simulink model "Project"  (R2018a)
settings: Solver=VariableStepAuto  StartTime=0  StopTime=1  FixedStep=Ts  RelTol=1e-3  AbsTol=1e-3
PreLoadFcn:
  | Ts=2e-6;
  | Ts_Control=100e-6;
undefined symbols (not defined in the file): Hydride, Metal, Nickel, Vnom_dc
libraries: powerlib x111, powerlib_extras x45, simulink x32, powerlib_meascontrol x13, dspswit3 x9, electricdrivelib x2, re_lib x2
(part 2 of 4)

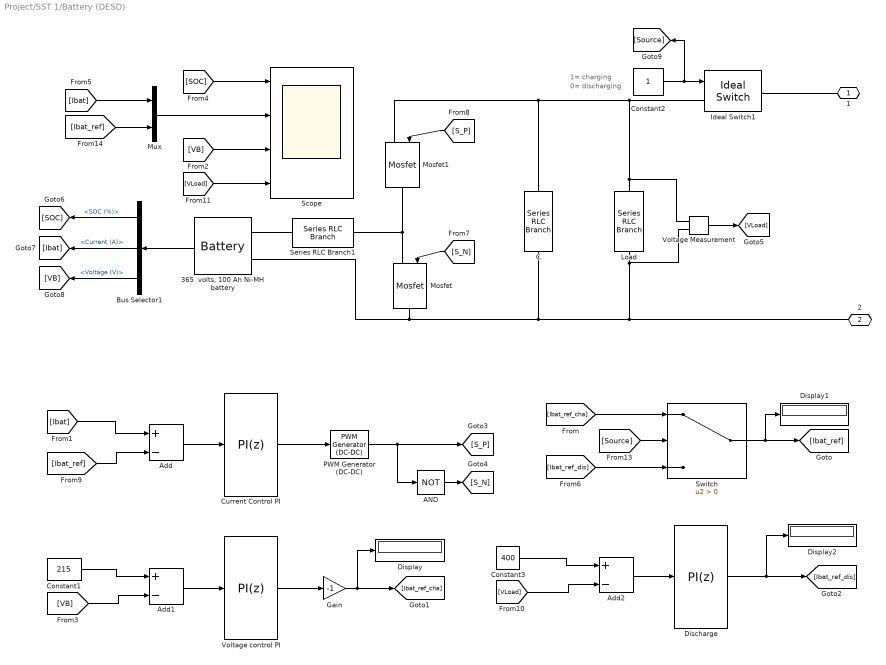
== system Project/SST 1/Battery (DESD) ==
  note: 1= charging
  note: 0= discharging
  "365  volts, 100 Ah Ni-MH battery" : electricdrivelib/Extra Sources/Battery  BatType=Nickel-Metal-Hydride  ShowTempParam=off  ThermalPreset=no  ShowAgeParam=off  NomV=365  NomQ=100  SOC=45  Batt_Tr=1  PresetModel=on  MaxQ=107.6923  MinV=273.75  FullV=429.9576  Dis_rate=20  R=0.0365  Normal_OP=96.1538  expZone="[395.9322            20]"  current=[6.5 13 32.5]  Units=Time  Tci=20  NomT=25  T2=0  MaxQ2=2.208  FullV2=3.45  Normal_OP2=2.8  expZone2="[3.22        0.23]"  Rca=0.6  ti=1000  Dp=0  Neq0=0  Tsim=1e6  Ta1=25  Qeol=5.4*0.9  Reol=0.013333*1.2  Char_age=[2.3478, 3]  Dis_age=[2.3478, 10]  N1=1500  N2=10500  N3=1000  N4=1400  Ta2=45  N5=950
      settings: SourceProductName=Simscape Electrical
  AND : Logic  Operator=NOT  AllPortsSameDT=off  OutDataTypeStr=boolean
  Add : Sum  Inputs=+-
  Add1 : Sum  Inputs=+-
  Add2 : Sum  Inputs=+-
  Bus Selector1 : BusSelector  OutputSignals=SOC (%),Current (A),Voltage (V)
  C : powerlib/Elements/Series RLC Branch  LConnTagsString=__new0  RConnTagsString=__new0  BranchType=RC  Resistance=0  Inductance=1e-3  SetiL0=off  InitialCurrent=0  Capacitance=1000e-6  Setx0=off  InitialVoltage=0  Measurements=None
      settings: SourceProductName=Simscape Electrical
  Constant1 : Constant  Value=215
  Constant2 : Constant
  Constant3 : Constant  Value=400
  Current Control PI : simulink/Continuous/PID Controller  Controller=PI  TimeDomain=Discrete-time  SampleTime=50e-6  IntegratorMethod=Forward Euler  FilterMethod=Forward Euler  Form=Parallel  UseFilter=on  ControllerParametersSource=internal  P=0.005  I=10  D=0  N=100  InitialConditionSource=internal  InitialConditionForIntegrator=0.54  InitialConditionForFilter=0  ExternalReset=none  LimitOutput=on  UpperSaturationLimit=0.95  LowerSaturationLimit=0  LinearizeAsGain=off  AntiWindupMode=none  Kb=1  TrackingMode=off  Kt=1  PParamMin=[]  PParamMax=[]  IParamMin=[]  IParamMax=[]  DParamMin=[]  DParamMax=[]  NParamMin=[]  NParamMax=[]  KbParamMin=[]  KbParamMax=[]  KtParamMin=[]  KtParamMax=[]  POutMin=[]  POutMax=[]  IOutMin=[]  IOutMax=[]  DOutMin=[]  DOutMax=[]  NOutMin=[]  NOutMax=[]  KbOutMin=[]  KbOutMax=[]  KtOutMin=[]  KtOutMax=[]  IntegratorOutMin=[]  IntegratorOutMax=[]  FilterOutMin=[]  FilterOutMax=[]  SumOutMin=[]  SumOutMax=[]  SumI1OutMin=[]  SumI1OutMax=[]  SumI2OutMin=[]  SumI2OutMax=[]  SumI3OutMin=[]  SumI3OutMax=[]  SumDOutMin=[]  SumDOutMax=[]  SaturationOutMin=[]  SaturationOutMax=[]  IntegratorContinuousStateAttributes=''  IntegratorStateMustResolveToSignalObject=off  IntegratorRTWStateStorageClass=Auto  FilterContinuousStateAttributes=''  FilterStateMustResolveToSignalObject=off  FilterRTWStateStorageClass=Auto  DifferentiatorICPrevScaledInput=0  DifferentiatorOutMin=[]  DifferentiatorOutMax=[]  FilterDiffOutCoefMin=[]  FilterDiffOutCoefMax=[]  SumDenOutMin=[]  SumDenOutMax=[]  SumNumOutMin=[]  SumNumOutMax=[]  ReciprocalOutMin=[]  ReciprocalOutMax=[]  DivideOutMin=[]  DivideOutMax=[]  TunerSelectOption=Transfer Function Based (PID Tuner App)
  Discharge : simulink/Continuous/PID Controller  Controller=PI  TimeDomain=Discrete-time  SampleTime=50e-6  IntegratorMethod=Forward Euler  FilterMethod=Forward Euler  Form=Parallel  UseFilter=on  ControllerParametersSource=internal  P=0.25  I=50  D=0  N=100  InitialConditionSource=internal  InitialConditionForIntegrator=0  InitialConditionForFilter=0  ExternalReset=none  LimitOutput=on  UpperSaturationLimit=12  LowerSaturationLimit=0  LinearizeAsGain=off  AntiWindupMode=none  Kb=1  TrackingMode=off  Kt=1  PParamMin=[]  PParamMax=[]  IParamMin=[]  IParamMax=[]  DParamMin=[]  DParamMax=[]  NParamMin=[]  NParamMax=[]  KbParamMin=[]  KbParamMax=[]  KtParamMin=[]  KtParamMax=[]  POutMin=[]  POutMax=[]  IOutMin=[]  IOutMax=[]  DOutMin=[]  DOutMax=[]  NOutMin=[]  NOutMax=[]  KbOutMin=[]  KbOutMax=[]  KtOutMin=[]  KtOutMax=[]  IntegratorOutMin=[]  IntegratorOutMax=[]  FilterOutMin=[]  FilterOutMax=[]  SumOutMin=[]  SumOutMax=[]  SumI1OutMin=[]  SumI1OutMax=[]  SumI2OutMin=[]  SumI2OutMax=[]  SumI3OutMin=[]  SumI3OutMax=[]  SumDOutMin=[]  SumDOutMax=[]  SaturationOutMin=[]  SaturationOutMax=[]  IntegratorContinuousStateAttributes=''  IntegratorStateMustResolveToSignalObject=off  IntegratorRTWStateStorageClass=Auto  FilterContinuousStateAttributes=''  FilterStateMustResolveToSignalObject=off  FilterRTWStateStorageClass=Auto  DifferentiatorICPrevScaledInput=0  DifferentiatorOutMin=[]  DifferentiatorOutMax=[]  FilterDiffOutCoefMin=[]  FilterDiffOutCoefMax=[]  SumDenOutMin=[]  SumDenOutMax=[]  SumNumOutMin=[]  SumNumOutMax=[]  ReciprocalOutMin=[]  ReciprocalOutMax=[]  DivideOutMin=[]  DivideOutMax=[]  TunerSelectOption=Transfer Function Based (PID Tuner App)
  Display : Display
  Display1 : Display
  Display2 : Display
  Gain : Gain  Gain=-1
  Ideal Switch1 : powerlib/Power Electronics/Ideal Switch  Ron=0.001  Lon=0  IC=0  Rs=1e5  Cs=inf  Measurements=off
      settings: SourceProductName=Simscape Electrical
  Load : powerlib/Elements/Series RLC Branch  LConnTagsString=__new0  RConnTagsString=__new0  BranchType=R  Resistance=10  Inductance=1e-3  SetiL0=off  InitialCurrent=0  Capacitance=1e-6  Setx0=off  InitialVoltage=0  Measurements=None
      settings: SourceProductName=Simscape Electrical
  Mosfet : powerlib/Power Electronics/Mosfet  Ron=0.1  Lon=0  Rd=0.01  Vfd=0  IC=0  Rs=1e5  Cs=inf  Measurements=off
      settings: SourceProductName=Simscape Electrical
  Mosfet1 : powerlib/Power Electronics/Mosfet  Ron=0.1  Lon=0  Rd=0.01  Vfd=0  IC=0  Rs=1e5  Cs=inf  Measurements=off
      settings: SourceProductName=Simscape Electrical
  Mux : Mux  Inputs=2
  PWM Generator (DC-DC) : powerlib_meascontrol/Pulse & Signal Generators/PWM Generator (DC-DC)  Fsw=10e3  Ts=5e-6
      settings: SourceProductName=Simscape Electrical
  Scope : Scope  NumInputPorts=4
  Series RLC Branch1 : powerlib/Elements/Series RLC Branch  LConnTagsString=__new0  RConnTagsString=__new0  BranchType=RL  Resistance=0.05  Inductance=5.76e-4  SetiL0=off  InitialCurrent=0  Capacitance=1e-6  Setx0=off  InitialVoltage=0  Measurements=None
      settings: SourceProductName=Simscape Electrical
  Switch : Switch  Criteria=u2 > Threshold
  Voltage Measurement : powerlib/Measurements/Voltage Measurement  PhasorSimulation=off  OutputType=Complex  PSBequivalent=0
      settings: SourceProductName=Simscape Electrical
  Voltage control PI : simulink/Continuous/PID Controller  Controller=PI  TimeDomain=Discrete-time  SampleTime=500e-6  IntegratorMethod=Forward Euler  FilterMethod=Forward Euler  Form=Parallel  UseFilter=on  ControllerParametersSource=internal  P=40  I=2000  D=0  N=100  InitialConditionSource=internal  InitialConditionForIntegrator=0  InitialConditionForFilter=0  ExternalReset=none  LimitOutput=on  UpperSaturationLimit=12  LowerSaturationLimit=0  LinearizeAsGain=off  AntiWindupMode=none  Kb=1  TrackingMode=off  Kt=1  PParamMin=[]  PParamMax=[]  IParamMin=[]  IParamMax=[]  DParamMin=[]  DParamMax=[]  NParamMin=[]  NParamMax=[]  KbParamMin=[]  KbParamMax=[]  KtParamMin=[]  KtParamMax=[]  POutMin=[]  POutMax=[]  IOutMin=[]  IOutMax=[]  DOutMin=[]  DOutMax=[]  NOutMin=[]  NOutMax=[]  KbOutMin=[]  KbOutMax=[]  KtOutMin=[]  KtOutMax=[]  IntegratorOutMin=[]  IntegratorOutMax=[]  FilterOutMin=[]  FilterOutMax=[]  SumOutMin=[]  SumOutMax=[]  SumI1OutMin=[]  SumI1OutMax=[]  SumI2OutMin=[]  SumI2OutMax=[]  SumI3OutMin=[]  SumI3OutMax=[]  SumDOutMin=[]  SumDOutMax=[]  SaturationOutMin=[]  SaturationOutMax=[]  IntegratorContinuousStateAttributes=''  IntegratorStateMustResolveToSignalObject=off  IntegratorRTWStateStorageClass=Auto  FilterContinuousStateAttributes=''  FilterStateMustResolveToSignalObject=off  FilterRTWStateStorageClass=Auto  DifferentiatorICPrevScaledInput=0  DifferentiatorOutMin=[]  DifferentiatorOutMax=[]  FilterDiffOutCoefMin=[]  FilterDiffOutCoefMax=[]  SumDenOutMin=[]  SumDenOutMax=[]  SumNumOutMin=[]  SumNumOutMax=[]  ReciprocalOutMin=[]  ReciprocalOutMax=[]  DivideOutMin=[]  DivideOutMax=[]  TunerSelectOption=Transfer Function Based (PID Tuner App)
  1 : PMIOPort  Side=Right
  2 : PMIOPort  Port=2  Side=Left
  wires:
  Current Control PI/1 -> PWM Generator (DC-DC)/1
  PWM Generator (DC-DC)/1 -> AND/1, [S_P]
  Bus Selector1/2 -> [Ibat]  "<Current (A)>"
  [SOC] -> Scope/1
  [S_N] -> Mosfet/1
  Discharge/1 -> Display2/1, [Ibat_ref_dis]
  [Ibat] -> Mux/1
  [Ibat_ref] -> Mux/2
  [VB] -> Add1/2
  "365  volts, 100 Ah Ni-MH battery"/1 -> Bus Selector1/1
  [VB] -> Scope/3
  Constant2/1 -> [Source], Ideal Switch1/1
  Bus Selector1/1 -> [SOC]  "<SOC (%)>"
  Add1/1 -> Voltage control PI/1
  Gain/1 -> Display/1, [Ibat_ref_cha]
  [S_P] -> Mosfet1/1
  [Ibat_ref_dis] -> Switch/3
  Voltage control PI/1 -> Gain/1
  [Ibat_ref] -> Add/2
  [Ibat] -> Add/1
  [VLoad] -> Add2/2
  Bus Selector1/3 -> [VB]  "<Voltage (V)>"
  Add/1 -> Current Control PI/1
  [VLoad] -> Scope/4
  Switch/1 -> [Ibat_ref], Display1/1
  Constant3/1 -> Add2/1
  AND/1 -> [S_N]
  [Source] -> Switch/2
  Mux/1 -> Scope/2
  Constant1/1 -> Add1/1
  [Ibat_ref_cha] -> Switch/1
  Add2/1 -> Discharge/1
  Voltage Measurement/1 -> [VLoad]
  connections:
  Ideal Switch1/LConn1 -- Load/RConn1 -- Voltage Measurement/LConn1 -- Mosfet1/LConn1 -- C/RConn1
  Load/LConn1 -- 2/RConn1 -- "365  volts, 100 Ah Ni-MH battery"/LConn2 -- Mosfet/RConn1 -- C/LConn1 -- Voltage Measurement/LConn2
  Series RLC Branch1/RConn1 -- Mosfet1/RConn1 -- Mosfet/LConn1
  "365  volts, 100 Ah Ni-MH battery"/LConn1 -- Series RLC Branch1/LConn1
  Ideal Switch1/RConn1 -- 1/RConn1

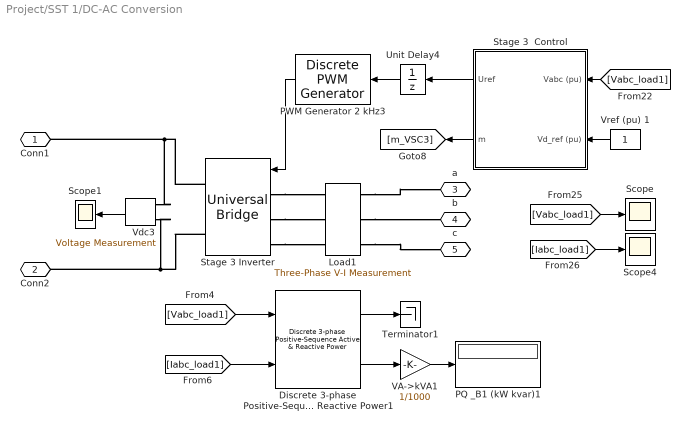
== system Project/SST 1/DC-AC Conversion ==
  Discrete 3-phase Positive-Sequence Active & Reactive Power1 : powerlib_extras/Discrete Measurements/Discrete 3-phase  Positive-Sequence  Active & Reactive Power  Freq=60  Par_Vinit=[0 0]  Par_Iinit=[0 0]  Ts=Ts
  Load1 : powerlib/Measurements/Three-Phase V-I Measurement  VoltageMeasurement=phase-to-phase  SetLabelV=on  LabelV=Vabc_load1  Vpu=off  VpuLL=off  CurrentMeasurement=yes  SetLabelI=on  LabelI=Iabc_load1  Ipu=off  Pbase=1e3  Vbase=380  OutputType=Magnitude  PhasorSimulation=off  PSBequivalent=0
  PQ _B1 (kW kvar)1 : Display
      settings: Decimation=2000
  PWM Generator 2 kHz3 : powerlib_extras/Discrete  Control Blocks/Discrete PWM Generator  GeneratorMode="3-arm  bridge (6 pulses)"  Fc=2000  Ts=Ts  Internal=off  mIndex=0.4  Freq=60  Phase=0
  Scope : Scope
  Scope1 : Scope
  Scope4 : Scope
  Stage 3 Inverter : powerlib/Power Electronics/Universal Bridge  Arms=3  SnubberResistance=1e5  SnubberCapacitance=inf  Device=IGBT / Diodes  Ron=1e-3  Lon=0  ForwardVoltages="[  0.0  0.0  ]"  ForwardVoltage=.8  GTOparameters=[ 1e-6 ,1e-6 ]  IGBTparameters="[ 0  0 ]"  Measurements=Device currents  Measurements_2=None  converterType=Rectifier
  "Stage 3  Control " : Subsystem  mask(Voltage Regulator){Kp=0.3, Ki=300, Vnom_load=380, Vnom_dc=680, Ts=Ts_Control}
      mask prompts: Kp "Proportional gain  Kp:"; Ki "Integral gain Ki:"; Vnom_load "Nominal load voltage (VrmsLL)"; Vnom_dc "Nominal DC bus voltage (V):"; Ts "Sample time (s) :"
  Terminator1 : Terminator
  Unit Delay4 : UnitDelay  SampleTime=Ts_Control
  VA->kVA1 : Gain  Gain=1/1000
  "Vdc3 " : powerlib/Measurements/Voltage Measurement  PhasorSimulation=off  OutputType=Complex  PSBequivalent=0
  Vref (pu) 1 : Constant
  Conn1 : PMIOPort  Side=Right
  Conn2 : PMIOPort  Port=2  Side=Right
  a : PMIOPort  Tag=PMCPort  Port=3  Side=Left
  " b" : PMIOPort  Tag=PMCPort  Port=4  Side=Left
  " c" : PMIOPort  Tag=PMCPort  Port=5  Side=Left
  wires:
  "Stage 3  Control "/2(m) -> [m_VSC3]
  Vref (pu) 1/1 -> "Stage 3  Control "/2(Vd_ref (pu))
  [Vabc_load1] -> "Stage 3  Control "/1(Vabc (pu))
  [Vabc_load1] -> Discrete 3-phase Positive-Sequence Active & Reactive Power1/1
  PWM Generator 2 kHz3/1 -> Stage 3 Inverter/1
  Unit Delay4/1 -> PWM Generator 2 kHz3/1
  VA->kVA1/1 -> PQ _B1 (kW kvar)1/1
  [Iabc_load1] -> Discrete 3-phase Positive-Sequence Active & Reactive Power1/2
  "Stage 3  Control "/1(Uref) -> Unit Delay4/1
  [Iabc_load1] -> Scope4/1
  [Vabc_load1] -> Scope/1
  Discrete 3-phase Positive-Sequence Active & Reactive Power1/2 -> VA->kVA1/1
  Discrete 3-phase Positive-Sequence Active & Reactive Power1/1 -> Terminator1/1
  "Vdc3 "/1 -> Scope1/1
  connections:
  Load1/RConn2 -- " b"/RConn1
  Load1/RConn3 -- " c"/RConn1
  Load1/RConn1 -- a/RConn1
  Stage 3 Inverter/LConn1 -- Load1/LConn1
  Stage 3 Inverter/LConn2 -- Load1/LConn2
  Stage 3 Inverter/LConn3 -- Load1/LConn3
  Stage 3 Inverter/RConn2 -- "Vdc3 "/LConn2 -- Conn2/RConn1
  Stage 3 Inverter/RConn1 -- "Vdc3 "/LConn1 -- Conn1/RConn1

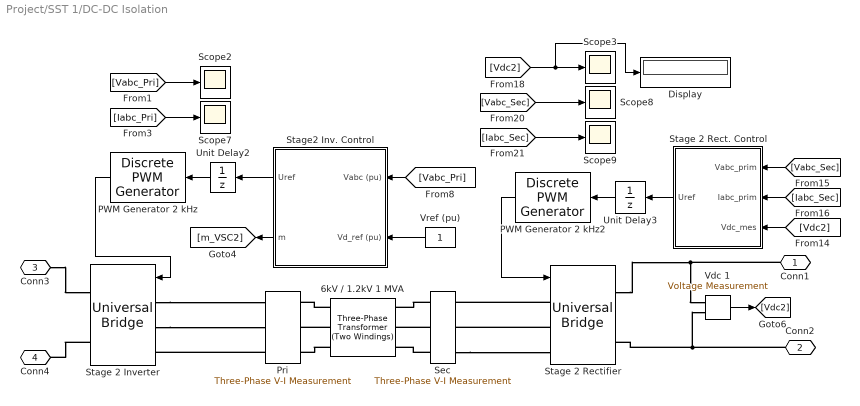
== system Project/SST 1/DC-DC Isolation ==
  6kV / 1.2kV 1 MVA : powerlib/Elements/Three-Phase Transformer (Two Windings)  Winding1Connection=Yg  Winding2Connection=Yg  CoreType=Three single-phase transformers  SetSaturation=off  Hysteresis=off  DataFile='hysteresis'  SetInitialFlux=off  Measurements=None  UNITS=pu  NominalPower=[ 1e6 , 60 ]  Winding1=[ 6e3 , 0.004 , 0.02 ]  Winding2=[ 1.2e3 , 0.004 , 0.02 ]  Rm=200  Lm=200  L0=0.5  Saturation="[ 0,0  ;  0.005,1.2  ;  1.0,1.4 ]"  InitialFluxes=[ 0.8 , -0.8 , 0.7 ]  MoreParameters=off  BreakLoop=off  DataType=off  TransfoNumber=0
  Display : Display
  PWM Generator 2 kHz : powerlib_extras/Discrete  Control Blocks/Discrete PWM Generator  GeneratorMode="3-arm  bridge (6 pulses)"  Fc=2000  Ts=Ts  Internal=off  mIndex=0.4  Freq=60  Phase=0
  PWM Generator 2 kHz2 : powerlib_extras/Discrete  Control Blocks/Discrete PWM Generator  GeneratorMode="3-arm  bridge (6 pulses)"  Fc=2000  Ts=Ts  Internal=off  mIndex=0.4  Freq=60  Phase=0
  Pri : powerlib/Measurements/Three-Phase V-I Measurement  VoltageMeasurement=phase-to-ground  SetLabelV=on  LabelV=Vabc_Pri  Vpu=off  VpuLL=off  CurrentMeasurement=yes  SetLabelI=on  LabelI=Iabc_Pri  Ipu=off  Pbase=1e3  Vbase=380  OutputType=Magnitude  PhasorSimulation=off  PSBequivalent=0
  Scope{2..3,7..9} (5 alike) : Scope
  Sec : powerlib/Measurements/Three-Phase V-I Measurement  VoltageMeasurement=phase-to-ground  SetLabelV=on  LabelV=Vabc_Sec  Vpu=off  VpuLL=off  CurrentMeasurement=yes  SetLabelI=on  LabelI=Iabc_Sec  Ipu=off  Pbase=100e6  Vbase=500e3  OutputType=Magnitude  PhasorSimulation=off  PSBequivalent=0
  Stage 2 Inverter : powerlib/Power Electronics/Universal Bridge  Arms=3  SnubberResistance=1e5  SnubberCapacitance=inf  Device=IGBT / Diodes  Ron=1e-3  Lon=0  ForwardVoltages="[  0.0  0.0  ]"  ForwardVoltage=.8  GTOparameters=[ 1e-6 ,1e-6 ]  IGBTparameters="[ 0  0 ]"  Measurements=None  Measurements_2=None  converterType=Rectifier
  Stage 2 Rectifier : powerlib/Power Electronics/Universal Bridge  Arms=3  SnubberResistance=1e5  SnubberCapacitance=inf  Device=IGBT / Diodes  Ron=1e-3  Lon=0  ForwardVoltages="[  0  0  ]"  ForwardVoltage=0  GTOparameters=[ 10e-6 , 20e-6 ]  IGBTparameters="[ 0  0  ]"  Measurements=None  Measurements_2=None  converterType=Rectifier
  Stage 2 Rect. Control : Subsystem  mask(VSC Main Controller){nom=[ 50e3  60 ], Vnom=[ 1.6e3 400 ], Vnom_dc=680, RLxfo=[0.008  0.04 ], RLchoke=[2e-3*(2*pi*60)/50   2e-3], K_VDCreg=[7  800], K_Ireg=[0.3 20]*1.5, Ts=Ts_Control}
      mask prompts: nom "Nominal power and frequency [ Pnom(VA)  Fnom(Hz) ]:"; Vnom "Nominal primary and secondary voltages (Vrms LL) [ Vnom_prim   Vnom_sec ]:"; Vnom_dc "Nominal DC bus voltage (V):"; RLxfo "Total transformer leakage impedance (pu/Pnom) [ Rxfo  Lxf ]"; RLchoke "Choke impedance [ R(ohm) L(H) ]"; K_VDCreg "VDC regultator gains [ Kp  Ki ]:"; K_Ireg "Current regulator gains [ Kp  Ki ]:"; Ts "Sample time"
      mask init: same as Project/SST 1/AC-DC Conversion/Stage1 Control
  "Stage2 Inv. Control " : Subsystem  mask(Voltage Regulator){Kp=0.3, Ki=300, Vnom_load=3.5e3, Vnom_dc=680, Ts=Ts_Control}
      mask prompts: Kp "Proportional gain  Kp:"; Ki "Integral gain Ki:"; Vnom_load "Nominal load voltage (VrmsLL)"; Vnom_dc "Nominal DC bus voltage (V):"; Ts "Sample time (s) :"
  Unit Delay2 : UnitDelay  SampleTime=Ts_Control
  Unit Delay3 : UnitDelay  SampleTime=Ts_Control
  Vdc 1 : powerlib/Measurements/Voltage Measurement  Tag=PoWeRsYsTeMmEaSuReMeNt  PhasorSimulation=off  OutputType=Magnitude  PSBequivalent=0
  "Vref (pu) " : Constant
  Conn1 : PMIOPort  Side=Left
  Conn2 : PMIOPort  Port=2  Side=Left
  Conn3 : PMIOPort  Port=3  Side=Right
  Conn4 : PMIOPort  Port=4  Side=Right
  wires:
  "Vref (pu) "/1 -> "Stage2 Inv. Control "/2(Vd_ref (pu))
  [Vdc2] -> Stage 2 Rect. Control/3(Vdc_mes)
  [Iabc_Sec] -> Scope9/1
  PWM Generator 2 kHz/1 -> Stage 2 Inverter/1
  Vdc 1/1 -> [Vdc2]
  [Vabc_Pri] -> Scope2/1
  [Iabc_Pri] -> Scope7/1
  [Vdc2] -> Display/1, Scope3/1
  [Vabc_Sec] -> Scope8/1
  "Stage2 Inv. Control "/2(m) -> [m_VSC2]
  PWM Generator 2 kHz2/1 -> Stage 2 Rectifier/1
  Stage 2 Rect. Control/1(Uref) -> Unit Delay3/1
  [Vabc_Pri] -> "Stage2 Inv. Control "/1(Vabc (pu))
  Unit Delay3/1 -> PWM Generator 2 kHz2/1
  [Vabc_Sec] -> Stage 2 Rect. Control/1(Vabc_prim)
  [Iabc_Sec] -> Stage 2 Rect. Control/2(Iabc_prim)
  "Stage2 Inv. Control "/1(Uref) -> Unit Delay2/1
  Unit Delay2/1 -> PWM Generator 2 kHz/1
  connections:
  Stage 2 Inverter/LConn2 -- Pri/LConn2
  Sec/LConn1 -- 6kV / 1.2kV 1 MVA/RConn1
  6kV / 1.2kV 1 MVA/LConn2 -- Pri/RConn2
  Stage 2 Rectifier/RConn2 -- Vdc 1/LConn2 -- Conn2/RConn1
  Stage 2 Inverter/LConn1 -- Pri/LConn1
  Stage 2 Rectifier/RConn1 -- Vdc 1/LConn1 -- Conn1/RConn1
  6kV / 1.2kV 1 MVA/LConn3 -- Pri/RConn3
  Sec/LConn2 -- 6kV / 1.2kV 1 MVA/RConn2
  6kV / 1.2kV 1 MVA/LConn1 -- Pri/RConn1
  Sec/LConn3 -- 6kV / 1.2kV 1 MVA/RConn3
  Pri/LConn3 -- Stage 2 Inverter/LConn3
  Stage 2 Inverter/RConn2 -- Conn4/RConn1
  Conn3/RConn1 -- Stage 2 Inverter/RConn1
  Sec/RConn3 -- Stage 2 Rectifier/LConn3
  Stage 2 Rectifier/LConn1 -- Sec/RConn1
  Stage 2 Rectifier/LConn2 -- Sec/RConn2

== system Project/SST 1/PV (DRER) ==
  Bus Selector1 : BusSelector  OutputSignals=V_PV,I_PV,I_diode
  C1 : powerlib/Elements/Series RLC Branch  LConnTagsString=__new0  RConnTagsString=__new0  BranchType=C  Resistance=1.0  Inductance=1.0  SetiL0=off  InitialCurrent=0  Capacitance=1800e-6  Setx0=off  InitialVoltage=Vnom_dc/2  Measurements=None
      settings: SourceProductName=Simscape Electrical
  Irradiance (W/m2) : powerlib_meascontrol/Pulse & Signal Generators/Stair Generator  t=[0, 0.4, 1.0]  e=[1, 1, 1]*1000  Ts=5e-6
      settings: SourceProductName=Simscape Electrical
  PV : Scope  NumInputPorts=3
  PV Array : re_lib/Solar/PV Array  Npar=88  Nser=5  PlotType=array @ 1000 W/m2 & specified temperatures  S_vec="[ 1000  500  100 ]"  Temp_C_vec="[ 45 25  ]"  ModuleName=SunPower SPR-415E-WHT-D  PlotWhenSelected=off  Pm=414.801  Ncell=128  Voc=85.3  Isc=6.09  Vm=72.9  Im=5.69  beta_Voc_pc=-0.229  alpha_Isc_pc=0.030706  beta_Voc=-0.19534  alpha_Isc=0.00187  IL=6.0978  I0=7.1712e-13  nI=0.87223  Rsh=419.7813  Rs=0.5371  BAL=on  Tc=1e-6  Tfilter=5e-5
      settings: SourceProductName=Simscape Electrical
      settings: AttributesFormatString=|
      | %<ModuleName>
      | %<Nser>-module string
      | %<Npar> parallel strings
  Rate Limiter : RateLimiter  RisingSlewLimit=6000  FallingSlewLimit=-6000  SampleTimeMode=inherited  InitialCondition=1000
  Saturation : Saturate  UpperLimit=55  LowerLimit=5
  Scope : Scope
  Temperature (Deg. C) : Constant  Value=45
  "Vdc " : powerlib/Measurements/Voltage Measurement  Tag=PoWeRsYsTeMmEaSuReMeNt  PhasorSimulation=off  OutputType=Magnitude  PSBequivalent=0
      settings: SourceProductName=Simscape Electrical
  1 : PMIOPort  Tag=PMCPort  Side=Left
  " 2" : PMIOPort  Tag=PMCPort  Port=2  Side=Left
  wires:
  Rate Limiter/1 -> PV Array/1
  Bus Selector1/1 -> PV/1  "<V_PV>"
  [meas_PV] -> Bus Selector1/1
  [Vdc_meas] -> Scope/1
  Bus Selector1/2 -> PV/2  "<I_PV>"
  Bus Selector1/3 -> PV/3  "<I_diode>"
  "Vdc "/1 -> [Vdc_meas]
  PV Array/1 -> [meas_PV]
  Temperature (Deg. C)/1 -> Saturation/1
  Saturation/1 -> PV Array/2
  Irradiance (W/m2)/1 -> Rate Limiter/1
  connections:
  C1/RConn1 -- PV Array/RConn2 -- " 2"/RConn1 -- "Vdc "/LConn2
  C1/LConn1 -- PV Array/RConn1 -- 1/RConn1 -- "Vdc "/LConn1

== system Project/SST 1/Switch ==
  In1 : Inport
  NOT : Logic  Operator=NOT  IconShape=distinctive  AllPortsSameDT=off  OutDataTypeStr=boolean
  PV Switch : powerlib/Power Electronics/Ideal Switch  Ron=0.001  Lon=0  IC=0  Rs=1e5  Cs=inf  Measurements=off
  SST Switch : powerlib/Power Electronics/Ideal Switch  Ron=0.001  Lon=0  IC=0  Rs=1e5  Cs=inf  Measurements=off
  PV : PMIOPort  Side=Left
  SST : PMIOPort  Port=2  Side=Left
  out : PMIOPort  Port=3  Side=Right
  wires:
  In1/1 -> SST Switch/1, NOT/1
  NOT/1 -> PV Switch/1
  connections:
  SST Switch/RConn1 -- PV Switch/RConn1 -- out/RConn1
  PV Switch/LConn1 -- PV/RConn1
  SST Switch/LConn1 -- SST/RConn1

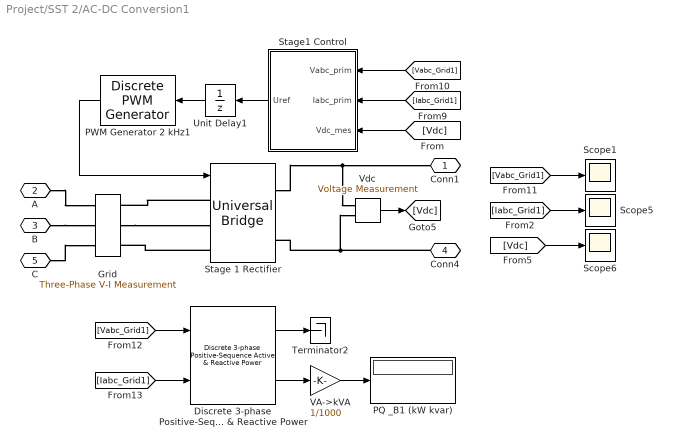
== system Project/SST 2/AC-DC Conversion1 ==
  Discrete 3-phase Positive-Sequence Active & Reactive Power : powerlib_extras/Discrete Measurements/Discrete 3-phase  Positive-Sequence  Active & Reactive Power  Freq=60  Par_Vinit=[0 0]  Par_Iinit=[0 0]  Ts=Ts
  Grid : powerlib/Measurements/Three-Phase V-I Measurement  VoltageMeasurement=phase-to-phase  SetLabelV=on  LabelV=Vabc_Grid1  Vpu=off  VpuLL=off  CurrentMeasurement=yes  SetLabelI=on  LabelI=Iabc_Grid1  Ipu=off  Pbase=100e6  Vbase=500e3  OutputType=Magnitude  PhasorSimulation=off  PSBequivalent=0
  PQ _B1 (kW kvar) : Display
      settings: Decimation=2000
  PWM Generator 2 kHz1 : powerlib_extras/Discrete  Control Blocks/Discrete PWM Generator  GeneratorMode="3-arm  bridge (6 pulses)"  Fc=2000  Ts=Ts  Internal=off  mIndex=0.4  Freq=60  Phase=0
  Scope1 : Scope
  Scope5 : Scope
  Scope6 : Scope
  Stage 1 Rectifier : powerlib/Power Electronics/Universal Bridge  Arms=3  SnubberResistance=1e5  SnubberCapacitance=inf  Device=IGBT / Diodes  Ron=1e-3  Lon=0  ForwardVoltages="[  0  0  ]"  ForwardVoltage=0  GTOparameters=[ 10e-6 , 20e-6 ]  IGBTparameters="[ 0  0  ]"  Measurements=None  Measurements_2=None  converterType=Rectifier
  Stage1 Control : Subsystem  mask(VSC Main Controller){nom=[ 50e3  60 ], Vnom=[ 4e3 1000 ], Vnom_dc=680, RLxfo=[0.008  0.04 ], RLchoke=[2e-3*(2*pi*60)/50   2e-3], K_VDCreg=[7  800], K_Ireg=[0.3 20]*1.5, Ts=Ts_Control}
      mask prompts: nom "Nominal power and frequency [ Pnom(VA)  Fnom(Hz) ]:"; Vnom "Nominal primary and secondary voltages (Vrms LL) [ Vnom_prim   Vnom_sec ]:"; Vnom_dc "Nominal DC bus voltage (V):"; RLxfo "Total transformer leakage impedance (pu/Pnom) [ Rxfo  Lxf ]"; RLchoke "Choke impedance [ R(ohm) L(H) ]"; K_VDCreg "VDC regultator gains [ Kp  Ki ]:"; K_Ireg "Current regulator gains [ Kp  Ki ]:"; Ts "Sample time"
      mask init: same as Project/SST 1/AC-DC Conversion/Stage1 Control
  Terminator2 : Terminator
  Unit Delay1 : UnitDelay  SampleTime=Ts_Control
  VA->kVA : Gain  Gain=1/1000
  "Vdc " : powerlib/Measurements/Voltage Measurement  Tag=PoWeRsYsTeMmEaSuReMeNt  PhasorSimulation=off  OutputType=Magnitude  PSBequivalent=0
  Conn1 : PMIOPort  Side=Right
  A : PMIOPort  Port=2  Side=Left
  B : PMIOPort  Port=3  Side=Left
  Conn4 : PMIOPort  Port=4  Side=Right
  C : PMIOPort  Port=5  Side=Left
  wires:
  [Vdc] -> Scope6/1
  [Vabc_Grid1] -> Discrete 3-phase Positive-Sequence Active & Reactive Power/1
  [Iabc_Grid1] -> Scope5/1
  [Iabc_Grid1] -> Stage1 Control/2(Iabc_prim)
  "Vdc "/1 -> [Vdc]
  [Iabc_Grid1] -> Discrete 3-phase Positive-Sequence Active & Reactive Power/2
  Stage1 Control/1(Uref) -> Unit Delay1/1
  Discrete 3-phase Positive-Sequence Active & Reactive Power/2 -> VA->kVA/1
  PWM Generator 2 kHz1/1 -> Stage 1 Rectifier/1
  VA->kVA/1 -> PQ _B1 (kW kvar)/1
  Discrete 3-phase Positive-Sequence Active & Reactive Power/1 -> Terminator2/1
  [Vdc] -> Stage1 Control/3(Vdc_mes)
  [Vabc_Grid1] -> Stage1 Control/1(Vabc_prim)
  Unit Delay1/1 -> PWM Generator 2 kHz1/1
  [Vabc_Grid1] -> Scope1/1
  connections:
  Stage 1 Rectifier/RConn2 -- "Vdc "/LConn2 -- Conn4/RConn1
  Stage 1 Rectifier/LConn1 -- Grid/RConn1
  Grid/RConn2 -- Stage 1 Rectifier/LConn2
  Stage 1 Rectifier/RConn1 -- "Vdc "/LConn1 -- Conn1/RConn1
  Stage 1 Rectifier/LConn3 -- Grid/RConn3
  C/RConn1 -- Grid/LConn3
  A/RConn1 -- Grid/LConn1
  B/RConn1 -- Grid/LConn2

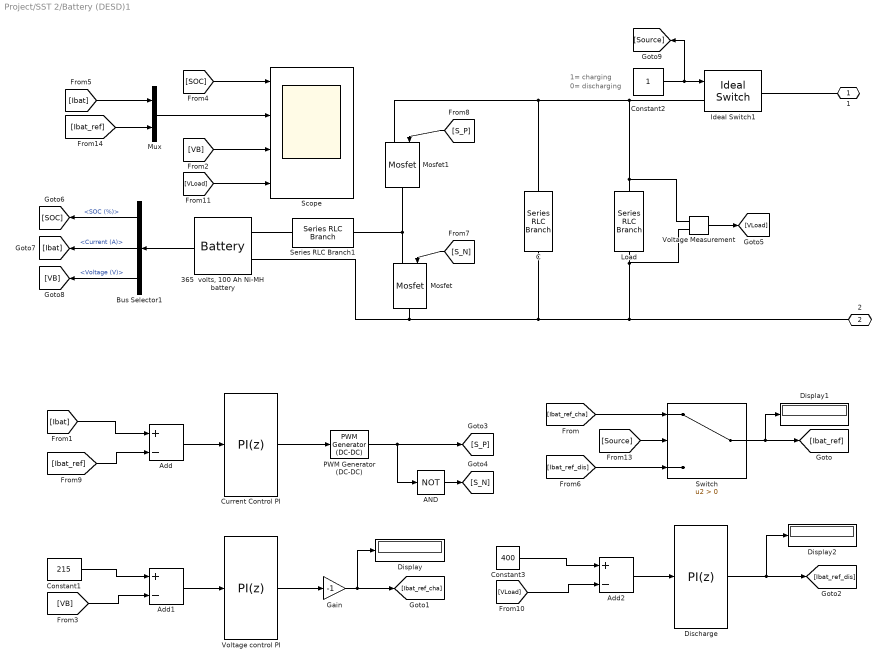
== system Project/SST 2/Battery (DESD)1 ==
  note: 1= charging
  note: 0= discharging
  "365  volts, 100 Ah Ni-MH battery" : electricdrivelib/Extra Sources/Battery  BatType=Nickel-Metal-Hydride  ShowTempParam=off  ThermalPreset=no  ShowAgeParam=off  NomV=365  NomQ=100  SOC=45  Batt_Tr=1  PresetModel=on  MaxQ=107.6923  MinV=273.75  FullV=429.9576  Dis_rate=20  R=0.0365  Normal_OP=96.1538  expZone="[395.9322            20]"  current=[6.5 13 32.5]  Units=Time  Tci=20  NomT=25  T2=0  MaxQ2=2.208  FullV2=3.45  Normal_OP2=2.8  expZone2="[3.22        0.23]"  Rca=0.6  ti=1000  Dp=0  Neq0=0  Tsim=1e6  Ta1=25  Qeol=5.4*0.9  Reol=0.013333*1.2  Char_age=[2.3478, 3]  Dis_age=[2.3478, 10]  N1=1500  N2=10500  N3=1000  N4=1400  Ta2=45  N5=950
      settings: SourceProductName=Simscape Electrical
  AND : Logic  Operator=NOT  AllPortsSameDT=off  OutDataTypeStr=boolean
  Add : Sum  Inputs=+-
  Add1 : Sum  Inputs=+-
  Add2 : Sum  Inputs=+-
  Bus Selector1 : BusSelector  OutputSignals=SOC (%),Current (A),Voltage (V)
  C : powerlib/Elements/Series RLC Branch  LConnTagsString=__new0  RConnTagsString=__new0  BranchType=RC  Resistance=0  Inductance=1e-3  SetiL0=off  InitialCurrent=0  Capacitance=1000e-6  Setx0=off  InitialVoltage=0  Measurements=None
      settings: SourceProductName=Simscape Electrical
  Constant1 : Constant  Value=215
  Constant2 : Constant
  Constant3 : Constant  Value=400
  Current Control PI : simulink/Continuous/PID Controller  Controller=PI  TimeDomain=Discrete-time  SampleTime=50e-6  IntegratorMethod=Forward Euler  FilterMethod=Forward Euler  Form=Parallel  UseFilter=on  ControllerParametersSource=internal  P=0.005  I=10  D=0  N=100  InitialConditionSource=internal  InitialConditionForIntegrator=0.54  InitialConditionForFilter=0  ExternalReset=none  LimitOutput=on  UpperSaturationLimit=0.95  LowerSaturationLimit=0  LinearizeAsGain=off  AntiWindupMode=none  Kb=1  TrackingMode=off  Kt=1  PParamMin=[]  PParamMax=[]  IParamMin=[]  IParamMax=[]  DParamMin=[]  DParamMax=[]  NParamMin=[]  NParamMax=[]  KbParamMin=[]  KbParamMax=[]  KtParamMin=[]  KtParamMax=[]  POutMin=[]  POutMax=[]  IOutMin=[]  IOutMax=[]  DOutMin=[]  DOutMax=[]  NOutMin=[]  NOutMax=[]  KbOutMin=[]  KbOutMax=[]  KtOutMin=[]  KtOutMax=[]  IntegratorOutMin=[]  IntegratorOutMax=[]  FilterOutMin=[]  FilterOutMax=[]  SumOutMin=[]  SumOutMax=[]  SumI1OutMin=[]  SumI1OutMax=[]  SumI2OutMin=[]  SumI2OutMax=[]  SumI3OutMin=[]  SumI3OutMax=[]  SumDOutMin=[]  SumDOutMax=[]  SaturationOutMin=[]  SaturationOutMax=[]  IntegratorContinuousStateAttributes=''  IntegratorStateMustResolveToSignalObject=off  IntegratorRTWStateStorageClass=Auto  FilterContinuousStateAttributes=''  FilterStateMustResolveToSignalObject=off  FilterRTWStateStorageClass=Auto  DifferentiatorICPrevScaledInput=0  DifferentiatorOutMin=[]  DifferentiatorOutMax=[]  FilterDiffOutCoefMin=[]  FilterDiffOutCoefMax=[]  SumDenOutMin=[]  SumDenOutMax=[]  SumNumOutMin=[]  SumNumOutMax=[]  ReciprocalOutMin=[]  ReciprocalOutMax=[]  DivideOutMin=[]  DivideOutMax=[]  TunerSelectOption=Transfer Function Based (PID Tuner App)
  Discharge : simulink/Continuous/PID Controller  Controller=PI  TimeDomain=Discrete-time  SampleTime=50e-6  IntegratorMethod=Forward Euler  FilterMethod=Forward Euler  Form=Parallel  UseFilter=on  ControllerParametersSource=internal  P=0.25  I=50  D=0  N=100  InitialConditionSource=internal  InitialConditionForIntegrator=0  InitialConditionForFilter=0  ExternalReset=none  LimitOutput=on  UpperSaturationLimit=12  LowerSaturationLimit=0  LinearizeAsGain=off  AntiWindupMode=none  Kb=1  TrackingMode=off  Kt=1  PParamMin=[]  PParamMax=[]  IParamMin=[]  IParamMax=[]  DParamMin=[]  DParamMax=[]  NParamMin=[]  NParamMax=[]  KbParamMin=[]  KbParamMax=[]  KtParamMin=[]  KtParamMax=[]  POutMin=[]  POutMax=[]  IOutMin=[]  IOutMax=[]  DOutMin=[]  DOutMax=[]  NOutMin=[]  NOutMax=[]  KbOutMin=[]  KbOutMax=[]  KtOutMin=[]  KtOutMax=[]  IntegratorOutMin=[]  IntegratorOutMax=[]  FilterOutMin=[]  FilterOutMax=[]  SumOutMin=[]  SumOutMax=[]  SumI1OutMin=[]  SumI1OutMax=[]  SumI2OutMin=[]  SumI2OutMax=[]  SumI3OutMin=[]  SumI3OutMax=[]  SumDOutMin=[]  SumDOutMax=[]  SaturationOutMin=[]  SaturationOutMax=[]  IntegratorContinuousStateAttributes=''  IntegratorStateMustResolveToSignalObject=off  IntegratorRTWStateStorageClass=Auto  FilterContinuousStateAttributes=''  FilterStateMustResolveToSignalObject=off  FilterRTWStateStorageClass=Auto  DifferentiatorICPrevScaledInput=0  DifferentiatorOutMin=[]  DifferentiatorOutMax=[]  FilterDiffOutCoefMin=[]  FilterDiffOutCoefMax=[]  SumDenOutMin=[]  SumDenOutMax=[]  SumNumOutMin=[]  SumNumOutMax=[]  ReciprocalOutMin=[]  ReciprocalOutMax=[]  DivideOutMin=[]  DivideOutMax=[]  TunerSelectOption=Transfer Function Based (PID Tuner App)
  Display : Display
  Display1 : Display
  Display2 : Display
  Gain : Gain  Gain=-1
  Ideal Switch1 : powerlib/Power Electronics/Ideal Switch  Ron=0.001  Lon=0  IC=0  Rs=1e5  Cs=inf  Measurements=off
      settings: SourceProductName=Simscape Electrical
  Load : powerlib/Elements/Series RLC Branch  LConnTagsString=__new0  RConnTagsString=__new0  BranchType=R  Resistance=10  Inductance=1e-3  SetiL0=off  InitialCurrent=0  Capacitance=1e-6  Setx0=off  InitialVoltage=0  Measurements=None
      settings: SourceProductName=Simscape Electrical
  Mosfet : powerlib/Power Electronics/Mosfet  Ron=0.1  Lon=0  Rd=0.01  Vfd=0  IC=0  Rs=1e5  Cs=inf  Measurements=off
      settings: SourceProductName=Simscape Electrical
  Mosfet1 : powerlib/Power Electronics/Mosfet  Ron=0.1  Lon=0  Rd=0.01  Vfd=0  IC=0  Rs=1e5  Cs=inf  Measurements=off
      settings: SourceProductName=Simscape Electrical
  Mux : Mux  Inputs=2
  PWM Generator (DC-DC) : powerlib_meascontrol/Pulse & Signal Generators/PWM Generator (DC-DC)  Fsw=10e3  Ts=5e-6
      settings: SourceProductName=Simscape Electrical
  Scope : Scope  NumInputPorts=4
  Series RLC Branch1 : powerlib/Elements/Series RLC Branch  LConnTagsString=__new0  RConnTagsString=__new0  BranchType=RL  Resistance=0.05  Inductance=5.76e-4  SetiL0=off  InitialCurrent=0  Capacitance=1e-6  Setx0=off  InitialVoltage=0  Measurements=None
      settings: SourceProductName=Simscape Electrical
  Switch : Switch  Criteria=u2 > Threshold
  Voltage Measurement : powerlib/Measurements/Voltage Measurement  PhasorSimulation=off  OutputType=Complex  PSBequivalent=0
      settings: SourceProductName=Simscape Electrical
  Voltage control PI : simulink/Continuous/PID Controller  Controller=PI  TimeDomain=Discrete-time  SampleTime=500e-6  IntegratorMethod=Forward Euler  FilterMethod=Forward Euler  Form=Parallel  UseFilter=on  ControllerParametersSource=internal  P=40  I=2000  D=0  N=100  InitialConditionSource=internal  InitialConditionForIntegrator=0  InitialConditionForFilter=0  ExternalReset=none  LimitOutput=on  UpperSaturationLimit=12  LowerSaturationLimit=0  LinearizeAsGain=off  AntiWindupMode=none  Kb=1  TrackingMode=off  Kt=1  PParamMin=[]  PParamMax=[]  IParamMin=[]  IParamMax=[]  DParamMin=[]  DParamMax=[]  NParamMin=[]  NParamMax=[]  KbParamMin=[]  KbParamMax=[]  KtParamMin=[]  KtParamMax=[]  POutMin=[]  POutMax=[]  IOutMin=[]  IOutMax=[]  DOutMin=[]  DOutMax=[]  NOutMin=[]  NOutMax=[]  KbOutMin=[]  KbOutMax=[]  KtOutMin=[]  KtOutMax=[]  IntegratorOutMin=[]  IntegratorOutMax=[]  FilterOutMin=[]  FilterOutMax=[]  SumOutMin=[]  SumOutMax=[]  SumI1OutMin=[]  SumI1OutMax=[]  SumI2OutMin=[]  SumI2OutMax=[]  SumI3OutMin=[]  SumI3OutMax=[]  SumDOutMin=[]  SumDOutMax=[]  SaturationOutMin=[]  SaturationOutMax=[]  IntegratorContinuousStateAttributes=''  IntegratorStateMustResolveToSignalObject=off  IntegratorRTWStateStorageClass=Auto  FilterContinuousStateAttributes=''  FilterStateMustResolveToSignalObject=off  FilterRTWStateStorageClass=Auto  DifferentiatorICPrevScaledInput=0  DifferentiatorOutMin=[]  DifferentiatorOutMax=[]  FilterDiffOutCoefMin=[]  FilterDiffOutCoefMax=[]  SumDenOutMin=[]  SumDenOutMax=[]  SumNumOutMin=[]  SumNumOutMax=[]  ReciprocalOutMin=[]  ReciprocalOutMax=[]  DivideOutMin=[]  DivideOutMax=[]  TunerSelectOption=Transfer Function Based (PID Tuner App)
  1 : PMIOPort  Side=Right
  2 : PMIOPort  Port=2  Side=Left
  wires:
  Current Control PI/1 -> PWM Generator (DC-DC)/1
  PWM Generator (DC-DC)/1 -> AND/1, [S_P]
  Bus Selector1/2 -> [Ibat]  "<Current (A)>"
  [SOC] -> Scope/1
  [S_N] -> Mosfet/1
  Discharge/1 -> Display2/1, [Ibat_ref_dis]
  [Ibat] -> Mux/1
  [Ibat_ref] -> Mux/2
  [VB] -> Add1/2
  "365  volts, 100 Ah Ni-MH battery"/1 -> Bus Selector1/1
  [VB] -> Scope/3
  Constant2/1 -> [Source], Ideal Switch1/1
  Bus Selector1/1 -> [SOC]  "<SOC (%)>"
  Add1/1 -> Voltage control PI/1
  Gain/1 -> Display/1, [Ibat_ref_cha]
  [S_P] -> Mosfet1/1
  [Ibat_ref_dis] -> Switch/3
  Voltage control PI/1 -> Gain/1
  [Ibat_ref] -> Add/2
  [Ibat] -> Add/1
  [VLoad] -> Add2/2
  Bus Selector1/3 -> [VB]  "<Voltage (V)>"
  Add/1 -> Current Control PI/1
  [VLoad] -> Scope/4
  Switch/1 -> [Ibat_ref], Display1/1
  Constant3/1 -> Add2/1
  AND/1 -> [S_N]
  [Source] -> Switch/2
  Mux/1 -> Scope/2
  Constant1/1 -> Add1/1
  [Ibat_ref_cha] -> Switch/1
  Add2/1 -> Discharge/1
  Voltage Measurement/1 -> [VLoad]
  connections:
  Ideal Switch1/LConn1 -- Load/RConn1 -- Voltage Measurement/LConn1 -- Mosfet1/LConn1 -- C/RConn1
  Load/LConn1 -- 2/RConn1 -- "365  volts, 100 Ah Ni-MH battery"/LConn2 -- Mosfet/RConn1 -- C/LConn1 -- Voltage Measurement/LConn2
  Series RLC Branch1/RConn1 -- Mosfet1/RConn1 -- Mosfet/LConn1
  "365  volts, 100 Ah Ni-MH battery"/LConn1 -- Series RLC Branch1/LConn1
  Ideal Switch1/RConn1 -- 1/RConn1

== system Project/SST 2/DC-AC Conversion1 ==
  Discrete 3-phase Positive-Sequence Active & Reactive Power1 : powerlib_extras/Discrete Measurements/Discrete 3-phase  Positive-Sequence  Active & Reactive Power  Freq=60  Par_Vinit=[0 0]  Par_Iinit=[0 0]  Ts=Ts
  Load1 : powerlib/Measurements/Three-Phase V-I Measurement  VoltageMeasurement=phase-to-phase  SetLabelV=on  LabelV=Vabc_load11  Vpu=off  VpuLL=off  CurrentMeasurement=yes  SetLabelI=on  LabelI=Iabc_load11  Ipu=off  Pbase=1e3  Vbase=380  OutputType=Magnitude  PhasorSimulation=off  PSBequivalent=0
  PQ _B1 (kW kvar)1 : Display
      settings: Decimation=2000
  PWM Generator 2 kHz3 : powerlib_extras/Discrete  Control Blocks/Discrete PWM Generator  GeneratorMode="3-arm  bridge (6 pulses)"  Fc=2000  Ts=Ts  Internal=off  mIndex=0.4  Freq=60  Phase=0
  Scope : Scope
  Scope1 : Scope
  Scope4 : Scope
  Stage 3 Inverter : powerlib/Power Electronics/Universal Bridge  Arms=3  SnubberResistance=1e5  SnubberCapacitance=inf  Device=IGBT / Diodes  Ron=1e-3  Lon=0  ForwardVoltages="[  0.0  0.0  ]"  ForwardVoltage=.8  GTOparameters=[ 1e-6 ,1e-6 ]  IGBTparameters="[ 0  0 ]"  Measurements=Device currents  Measurements_2=None  converterType=Rectifier
  "Stage 3  Control " : Subsystem  mask(Voltage Regulator){Kp=0.3, Ki=300, Vnom_load=380, Vnom_dc=680, Ts=Ts_Control}
      mask prompts: Kp "Proportional gain  Kp:"; Ki "Integral gain Ki:"; Vnom_load "Nominal load voltage (VrmsLL)"; Vnom_dc "Nominal DC bus voltage (V):"; Ts "Sample time (s) :"
  Terminator1 : Terminator
  Unit Delay4 : UnitDelay  SampleTime=Ts_Control
  VA->kVA1 : Gain  Gain=1/1000
  "Vdc3 " : powerlib/Measurements/Voltage Measurement  PhasorSimulation=off  OutputType=Complex  PSBequivalent=0
  Vref (pu) 1 : Constant
  Conn1 : PMIOPort  Side=Right
  Conn2 : PMIOPort  Port=2  Side=Right
  a : PMIOPort  Tag=PMCPort  Port=3  Side=Left
  " b" : PMIOPort  Tag=PMCPort  Port=4  Side=Left
  " c" : PMIOPort  Tag=PMCPort  Port=5  Side=Left
  wires:
  "Stage 3  Control "/2(m) -> [m_VSC3]
  Vref (pu) 1/1 -> "Stage 3  Control "/2(Vd_ref (pu))
  [Vabc_load11] -> "Stage 3  Control "/1(Vabc (pu))
  [Vabc_load11] -> Discrete 3-phase Positive-Sequence Active & Reactive Power1/1
  PWM Generator 2 kHz3/1 -> Stage 3 Inverter/1
  Unit Delay4/1 -> PWM Generator 2 kHz3/1
  VA->kVA1/1 -> PQ _B1 (kW kvar)1/1
  [Iabc_load11] -> Discrete 3-phase Positive-Sequence Active & Reactive Power1/2
  "Stage 3  Control "/1(Uref) -> Unit Delay4/1
  [Iabc_load11] -> Scope4/1
  [Vabc_load11] -> Scope/1
  Discrete 3-phase Positive-Sequence Active & Reactive Power1/2 -> VA->kVA1/1
  Discrete 3-phase Positive-Sequence Active & Reactive Power1/1 -> Terminator1/1
  "Vdc3 "/1 -> Scope1/1
  connections:
  Load1/RConn2 -- " b"/RConn1
  Load1/RConn3 -- " c"/RConn1
  Load1/RConn1 -- a/RConn1
  Stage 3 Inverter/LConn1 -- Load1/LConn1
  Stage 3 Inverter/LConn2 -- Load1/LConn2
  Stage 3 Inverter/LConn3 -- Load1/LConn3
  Stage 3 Inverter/RConn2 -- "Vdc3 "/LConn2 -- Conn2/RConn1
  Stage 3 Inverter/RConn1 -- "Vdc3 "/LConn1 -- Conn1/RConn1

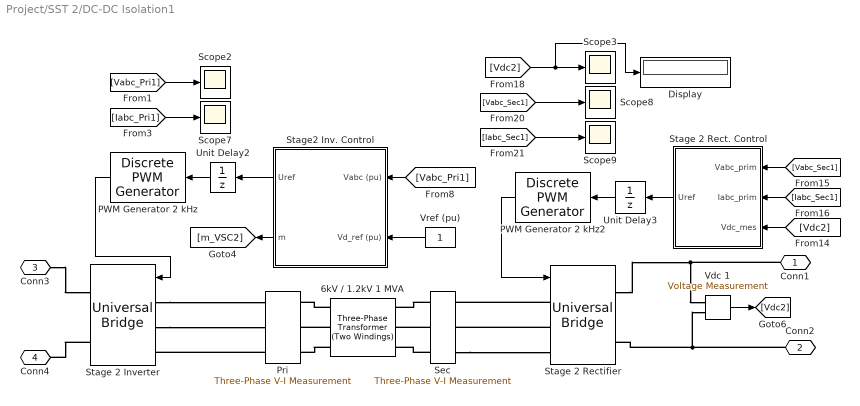
== system Project/SST 2/DC-DC Isolation1 ==
  6kV / 1.2kV 1 MVA : powerlib/Elements/Three-Phase Transformer (Two Windings)  Winding1Connection=Yg  Winding2Connection=Yg  CoreType=Three single-phase transformers  SetSaturation=off  Hysteresis=off  DataFile='hysteresis'  SetInitialFlux=off  Measurements=None  UNITS=pu  NominalPower=[ 1e6 , 60 ]  Winding1=[ 6e3 , 0.004 , 0.02 ]  Winding2=[ 1.2e3 , 0.004 , 0.02 ]  Rm=200  Lm=200  L0=0.5  Saturation="[ 0,0  ;  0.005,1.2  ;  1.0,1.4 ]"  InitialFluxes=[ 0.8 , -0.8 , 0.7 ]  MoreParameters=off  BreakLoop=off  DataType=off  TransfoNumber=0
  Display : Display
  PWM Generator 2 kHz : powerlib_extras/Discrete  Control Blocks/Discrete PWM Generator  GeneratorMode="3-arm  bridge (6 pulses)"  Fc=2000  Ts=Ts  Internal=off  mIndex=0.4  Freq=60  Phase=0
  PWM Generator 2 kHz2 : powerlib_extras/Discrete  Control Blocks/Discrete PWM Generator  GeneratorMode="3-arm  bridge (6 pulses)"  Fc=2000  Ts=Ts  Internal=off  mIndex=0.4  Freq=60  Phase=0
  Pri : powerlib/Measurements/Three-Phase V-I Measurement  VoltageMeasurement=phase-to-ground  SetLabelV=on  LabelV=Vabc_Pri1  Vpu=off  VpuLL=off  CurrentMeasurement=yes  SetLabelI=on  LabelI=Iabc_Pri1  Ipu=off  Pbase=1e3  Vbase=380  OutputType=Magnitude  PhasorSimulation=off  PSBequivalent=0
  Scope{2..3,7..9} (5 alike) : Scope
  Sec : powerlib/Measurements/Three-Phase V-I Measurement  VoltageMeasurement=phase-to-ground  SetLabelV=on  LabelV=Vabc_Sec1  Vpu=off  VpuLL=off  CurrentMeasurement=yes  SetLabelI=on  LabelI=Iabc_Sec1  Ipu=off  Pbase=100e6  Vbase=500e3  OutputType=Magnitude  PhasorSimulation=off  PSBequivalent=0
  Stage 2 Inverter : powerlib/Power Electronics/Universal Bridge  Arms=3  SnubberResistance=1e5  SnubberCapacitance=inf  Device=IGBT / Diodes  Ron=1e-3  Lon=0  ForwardVoltages="[  0.0  0.0  ]"  ForwardVoltage=.8  GTOparameters=[ 1e-6 ,1e-6 ]  IGBTparameters="[ 0  0 ]"  Measurements=None  Measurements_2=None  converterType=Rectifier
  Stage 2 Rectifier : powerlib/Power Electronics/Universal Bridge  Arms=3  SnubberResistance=1e5  SnubberCapacitance=inf  Device=IGBT / Diodes  Ron=1e-3  Lon=0  ForwardVoltages="[  0  0  ]"  ForwardVoltage=0  GTOparameters=[ 10e-6 , 20e-6 ]  IGBTparameters="[ 0  0  ]"  Measurements=None  Measurements_2=None  converterType=Rectifier
  Stage 2 Rect. Control : Subsystem  mask(VSC Main Controller){nom=[ 50e3  60 ], Vnom=[ 1.6e3 400 ], Vnom_dc=680, RLxfo=[0.008  0.04 ], RLchoke=[2e-3*(2*pi*60)/50   2e-3], K_VDCreg=[7  800], K_Ireg=[0.3 20]*1.5, Ts=Ts_Control}
      mask prompts: nom "Nominal power and frequency [ Pnom(VA)  Fnom(Hz) ]:"; Vnom "Nominal primary and secondary voltages (Vrms LL) [ Vnom_prim   Vnom_sec ]:"; Vnom_dc "Nominal DC bus voltage (V):"; RLxfo "Total transformer leakage impedance (pu/Pnom) [ Rxfo  Lxf ]"; RLchoke "Choke impedance [ R(ohm) L(H) ]"; K_VDCreg "VDC regultator gains [ Kp  Ki ]:"; K_Ireg "Current regulator gains [ Kp  Ki ]:"; Ts "Sample time"
      mask init: same as Project/SST 1/AC-DC Conversion/Stage1 Control
  "Stage2 Inv. Control " : Subsystem  mask(Voltage Regulator){Kp=0.3, Ki=300, Vnom_load=3.5e3, Vnom_dc=680, Ts=Ts_Control}
      mask prompts: Kp "Proportional gain  Kp:"; Ki "Integral gain Ki:"; Vnom_load "Nominal load voltage (VrmsLL)"; Vnom_dc "Nominal DC bus voltage (V):"; Ts "Sample time (s) :"
  Unit Delay2 : UnitDelay  SampleTime=Ts_Control
  Unit Delay3 : UnitDelay  SampleTime=Ts_Control
  Vdc 1 : powerlib/Measurements/Voltage Measurement  Tag=PoWeRsYsTeMmEaSuReMeNt  PhasorSimulation=off  OutputType=Magnitude  PSBequivalent=0
  "Vref (pu) " : Constant
  Conn1 : PMIOPort  Side=Left
  Conn2 : PMIOPort  Port=2  Side=Left
  Conn3 : PMIOPort  Port=3  Side=Right
  Conn4 : PMIOPort  Port=4  Side=Right
  wires:
  "Vref (pu) "/1 -> "Stage2 Inv. Control "/2(Vd_ref (pu))
  [Vdc2] -> Stage 2 Rect. Control/3(Vdc_mes)
  [Iabc_Sec1] -> Scope9/1
  PWM Generator 2 kHz/1 -> Stage 2 Inverter/1
  Vdc 1/1 -> [Vdc2]
  [Vabc_Pri1] -> Scope2/1
  [Iabc_Pri1] -> Scope7/1
  [Vdc2] -> Display/1, Scope3/1
  [Vabc_Sec1] -> Scope8/1
  "Stage2 Inv. Control "/2(m) -> [m_VSC2]
  PWM Generator 2 kHz2/1 -> Stage 2 Rectifier/1
  Stage 2 Rect. Control/1(Uref) -> Unit Delay3/1
  [Vabc_Pri1] -> "Stage2 Inv. Control "/1(Vabc (pu))
  Unit Delay3/1 -> PWM Generator 2 kHz2/1
  [Vabc_Sec1] -> Stage 2 Rect. Control/1(Vabc_prim)
  [Iabc_Sec1] -> Stage 2 Rect. Control/2(Iabc_prim)
  "Stage2 Inv. Control "/1(Uref) -> Unit Delay2/1
  Unit Delay2/1 -> PWM Generator 2 kHz/1
  connections:
  Stage 2 Inverter/LConn2 -- Pri/LConn2
  Sec/LConn1 -- 6kV / 1.2kV 1 MVA/RConn1
  6kV / 1.2kV 1 MVA/LConn2 -- Pri/RConn2
  Stage 2 Rectifier/RConn2 -- Vdc 1/LConn2 -- Conn2/RConn1
  Stage 2 Inverter/LConn1 -- Pri/LConn1
  Stage 2 Rectifier/RConn1 -- Vdc 1/LConn1 -- Conn1/RConn1
  6kV / 1.2kV 1 MVA/LConn3 -- Pri/RConn3
  Sec/LConn2 -- 6kV / 1.2kV 1 MVA/RConn2
  6kV / 1.2kV 1 MVA/LConn1 -- Pri/RConn1
  Sec/LConn3 -- 6kV / 1.2kV 1 MVA/RConn3
  Pri/LConn3 -- Stage 2 Inverter/LConn3
  Stage 2 Inverter/RConn2 -- Conn4/RConn1
  Conn3/RConn1 -- Stage 2 Inverter/RConn1
  Sec/RConn3 -- Stage 2 Rectifier/LConn3
  Stage 2 Rectifier/LConn1 -- Sec/RConn1
  Stage 2 Rectifier/LConn2 -- Sec/RConn2

== system Project/SST 2/PV (DRER)1 ==
  Bus Selector1 : BusSelector  OutputSignals=V_PV,I_PV,I_diode
  C1 : powerlib/Elements/Series RLC Branch  LConnTagsString=__new0  RConnTagsString=__new0  BranchType=C  Resistance=1.0  Inductance=1.0  SetiL0=off  InitialCurrent=0  Capacitance=1800e-6  Setx0=off  InitialVoltage=Vnom_dc/2  Measurements=None
      settings: SourceProductName=Simscape Electrical
  Irradiance (W/m2) : powerlib_meascontrol/Pulse & Signal Generators/Stair Generator  t=[0, 0.4, 1.0]  e=[1, 1, 1]*1000  Ts=5e-6
      settings: SourceProductName=Simscape Electrical
  PV : Scope  NumInputPorts=3
  PV Array : re_lib/Solar/PV Array  Npar=88  Nser=5  PlotType=array @ 1000 W/m2 & specified temperatures  S_vec="[ 1000  500  100 ]"  Temp_C_vec="[ 45 25  ]"  ModuleName=SunPower SPR-415E-WHT-D  PlotWhenSelected=off  Pm=414.801  Ncell=128  Voc=85.3  Isc=6.09  Vm=72.9  Im=5.69  beta_Voc_pc=-0.229  alpha_Isc_pc=0.030706  beta_Voc=-0.19534  alpha_Isc=0.00187  IL=6.0978  I0=7.1712e-13  nI=0.87223  Rsh=419.7813  Rs=0.5371  BAL=on  Tc=1e-6  Tfilter=5e-5
      settings: SourceProductName=Simscape Electrical
      settings: AttributesFormatString=|
      | %<ModuleName>
      | %<Nser>-module string
      | %<Npar> parallel strings
  Rate Limiter : RateLimiter  RisingSlewLimit=6000  FallingSlewLimit=-6000  SampleTimeMode=inherited  InitialCondition=1000
  Saturation : Saturate  UpperLimit=55  LowerLimit=5
  Scope : Scope
  Temperature (Deg. C) : Constant  Value=45
  "Vdc " : powerlib/Measurements/Voltage Measurement  Tag=PoWeRsYsTeMmEaSuReMeNt  PhasorSimulation=off  OutputType=Magnitude  PSBequivalent=0
      settings: SourceProductName=Simscape Electrical
  1 : PMIOPort  Tag=PMCPort  Side=Left
  " 2" : PMIOPort  Tag=PMCPort  Port=2  Side=Left
  wires:
  Rate Limiter/1 -> PV Array/1
  Bus Selector1/1 -> PV/1  "<V_PV>"
  [meas_PV] -> Bus Selector1/1
  [Vdc_meas] -> Scope/1
  Bus Selector1/2 -> PV/2  "<I_PV>"
  Bus Selector1/3 -> PV/3  "<I_diode>"
  "Vdc "/1 -> [Vdc_meas]
  PV Array/1 -> [meas_PV]
  Temperature (Deg. C)/1 -> Saturation/1
  Saturation/1 -> PV Array/2
  Irradiance (W/m2)/1 -> Rate Limiter/1
  connections:
  C1/RConn1 -- PV Array/RConn2 -- " 2"/RConn1 -- "Vdc "/LConn2
  C1/LConn1 -- PV Array/RConn1 -- 1/RConn1 -- "Vdc "/LConn1

== system Project/SST 2/Switch1 ==
  In1 : Inport
  NOT : Logic  Operator=NOT  IconShape=distinctive  AllPortsSameDT=off  OutDataTypeStr=boolean
  PV Switch : powerlib/Power Electronics/Ideal Switch  Ron=0.001  Lon=0  IC=0  Rs=1e5  Cs=inf  Measurements=off
  SST Switch : powerlib/Power Electronics/Ideal Switch  Ron=0.001  Lon=0  IC=0  Rs=1e5  Cs=inf  Measurements=off
  PV : PMIOPort  Side=Left
  SST : PMIOPort  Port=2  Side=Left
  out : PMIOPort  Port=3  Side=Right
  wires:
  In1/1 -> SST Switch/1, NOT/1
  NOT/1 -> PV Switch/1
  connections:
  SST Switch/RConn1 -- PV Switch/RConn1 -- out/RConn1
  PV Switch/LConn1 -- PV/RConn1
  SST Switch/LConn1 -- SST/RConn1

== system Project/PROTECTION 1/overcurrent relay1/Main Relay ==
  note: ca.culating peak
  "Three phase actual currents " : Inport
  "CT ratio " : Inport  Port=2
  Compare To Constant : simulink/Logic and Bit Operations/Compare To Constant  relop=<=  const=60  OutDataTypeStr=uint8  ZeroCross=off
  Compare To Zero : simulink/Logic and Bit Operations/Compare To Zero  relop=<=  OutDataTypeStr=uint8  ZeroCross=off
  Constant : Constant
  Data Type Conversion : DataTypeConversion  OutDataTypeStr=double
  Divide : Product  Inputs=*/
  Gain : Gain  Gain=sqrt(2)
  Logical Operator : Logic  Operator=XOR  AllPortsSameDT=off  OutDataTypeStr=boolean
  RMS1 : powerlib_extras/Measurements/RMS  f1=50
  Scope{2..5} (4 alike) : Scope
  AR signal : Outport
  wires:
  "Three phase actual currents "/1 -> RMS1/1
  "CT ratio "/1 -> Divide/2
  RMS1/1 -> Gain/1
  Gain/1 -> Divide/1
  Divide/1 -> Compare To Constant/1, Scope4/1  "Ip"
  Compare To Constant/1 -> Scope5/1, Compare To Zero/1
  Constant/1 -> Logical Operator/2
  Data Type Conversion/1 -> AR signal/1
  Logical Operator/1 -> Data Type Conversion/1, Scope2/1
  Compare To Zero/1 -> Scope3/1, Logical Operator/1

== system Project/PROTECTION 1/overcurrent relay2/Main Relay ==
  note: ca.culating peak
  "Three phase actual currents " : Inport
  "CT ratio " : Inport  Port=2
  Compare To Constant : simulink/Logic and Bit Operations/Compare To Constant  relop=<=  const=60  OutDataTypeStr=uint8  ZeroCross=off
  Compare To Zero : simulink/Logic and Bit Operations/Compare To Zero  relop=<=  OutDataTypeStr=uint8  ZeroCross=off
  Constant : Constant
  Data Type Conversion : DataTypeConversion  OutDataTypeStr=double
  Divide : Product  Inputs=*/
  Gain : Gain  Gain=sqrt(2)
  Logical Operator : Logic  Operator=XOR  AllPortsSameDT=off  OutDataTypeStr=boolean
  RMS1 : powerlib_extras/Measurements/RMS  f1=50
  Scope{2..5} (4 alike) : Scope
  AR signal : Outport
  wires:
  Compare To Zero/1 -> Logical Operator/1, Scope3/1
  Logical Operator/1 -> Scope2/1, Data Type Conversion/1
  Data Type Conversion/1 -> AR signal/1
  Constant/1 -> Logical Operator/2
  Compare To Constant/1 -> Compare To Zero/1, Scope5/1
  Divide/1 -> Scope4/1, Compare To Constant/1  "Ip"
  Gain/1 -> Divide/1
  RMS1/1 -> Gain/1
  "CT ratio "/1 -> Divide/2
  "Three phase actual currents "/1 -> RMS1/1

== system Project/PROTECTION 1/overcurrent relay3/Main Relay ==
  note: ca.culating peak
  "Three phase actual currents " : Inport
  "CT ratio " : Inport  Port=2
  Compare To Constant : simulink/Logic and Bit Operations/Compare To Constant  relop=<=  const=60  OutDataTypeStr=uint8  ZeroCross=off
  Compare To Zero : simulink/Logic and Bit Operations/Compare To Zero  relop=<=  OutDataTypeStr=uint8  ZeroCross=off
  Constant : Constant
  Data Type Conversion : DataTypeConversion  OutDataTypeStr=double
  Divide : Product  Inputs=*/
  Gain : Gain  Gain=sqrt(2)
  Logical Operator : Logic  Operator=XOR  AllPortsSameDT=off  OutDataTypeStr=boolean
  RMS1 : powerlib_extras/Measurements/RMS  f1=50
  Scope{2..5} (4 alike) : Scope
  AR signal : Outport
  wires:
  Compare To Zero/1 -> Logical Operator/1, Scope3/1
  Logical Operator/1 -> Scope2/1, Data Type Conversion/1
  Data Type Conversion/1 -> AR signal/1
  Constant/1 -> Logical Operator/2
  Compare To Constant/1 -> Compare To Zero/1, Scope5/1
  Divide/1 -> Scope4/1, Compare To Constant/1  "Ip"
  Gain/1 -> Divide/1
  RMS1/1 -> Gain/1
  "CT ratio "/1 -> Divide/2
  "Three phase actual currents "/1 -> RMS1/1

== system Project/PROTECTION 2/overcurrent relay1/Main Relay ==
  note: ca.culating peak
  "Three phase actual currents " : Inport
  "CT ratio " : Inport  Port=2
  Compare To Constant : simulink/Logic and Bit Operations/Compare To Constant  relop=<=  const=60  OutDataTypeStr=uint8  ZeroCross=off
  Compare To Zero : simulink/Logic and Bit Operations/Compare To Zero  relop=<=  OutDataTypeStr=uint8  ZeroCross=off
  Constant : Constant
  Data Type Conversion : DataTypeConversion  OutDataTypeStr=double
  Divide : Product  Inputs=*/
  Gain : Gain  Gain=sqrt(2)
  Logical Operator : Logic  Operator=XOR  AllPortsSameDT=off  OutDataTypeStr=boolean
  RMS1 : powerlib_extras/Measurements/RMS  f1=50
  Scope{2..5} (4 alike) : Scope
  AR signal : Outport
  wires:
  "Three phase actual currents "/1 -> RMS1/1
  "CT ratio "/1 -> Divide/2
  RMS1/1 -> Gain/1
  Gain/1 -> Divide/1
  Divide/1 -> Compare To Constant/1, Scope4/1  "Ip"
  Compare To Constant/1 -> Scope5/1, Compare To Zero/1
  Constant/1 -> Logical Operator/2
  Data Type Conversion/1 -> AR signal/1
  Logical Operator/1 -> Data Type Conversion/1, Scope2/1
  Compare To Zero/1 -> Scope3/1, Logical Operator/1
